simulink model "RobotAndBall"  (R2019b)
settings: Solver=VariableStepAuto  StartTime=0.0  StopTime=30  MaxStep=updateFrequency  RelTol=1e-3
values from neighbouring files (symbols this model uses):
  g = bTraj.GoalOnRight    [Launch_Game_TwoRobots.m]
  pOpponentSidePoint = [2.4;0;0.02]'    [Launch_Game_TwoRobots.m]
  Robot1 = RobotPlayer2(initialQ,TransMat1,DistToTable,'Left')    [Launch_Game_TwoRobots.m]
undefined symbols (not defined in the file or in its folder): Ball, Contact_Forces, currentTime, Environment, Net, Robots, Table, tHit, wayPoints, X, Y, Z
libraries: sm_lib x217, nesl_utility x89, Contact_Forces_Lib x8, robotmaniplib x8, Parts_Lib x6, Multibody_Parts_Lib x2, OpenManipulatorLib x1
(part 3 of 7)

== system RobotAndBall/failTryToPredictTraj ==
  In1 : Inport
  In2 : Inport  Port=2
  Append : MATLAB Function  TreatAsAtomicUnit=on
  Clock : Clock
  MATLAB Function : MATLAB Function  TreatAsAtomicUnit=on
  Subsystem : Subsystem
  Subsystem1 : Subsystem
  Subsystem3 : Subsystem
  Terminator : Terminator
  wires:
  In2/1 -> Append/4(Pnew)
  Append/2(Vout) -> MATLAB Function/2(V), Subsystem3/1(In1)
  MATLAB Function/1(aa) -> Terminator/1
  Clock/1 -> MATLAB Function/4(t)
  Append/3(Nout) -> MATLAB Function/3(N), Subsystem/1(In1)
  Append/1(Pout) -> Subsystem1/1(In1), MATLAB Function/1(P)
  Subsystem3/1(Out1) -> Append/1(V)
  Subsystem/1(Out1) -> Append/5(N)
  Subsystem1/1(Out1) -> Append/3(P)
  In1/1 -> Append/2(Vnew)

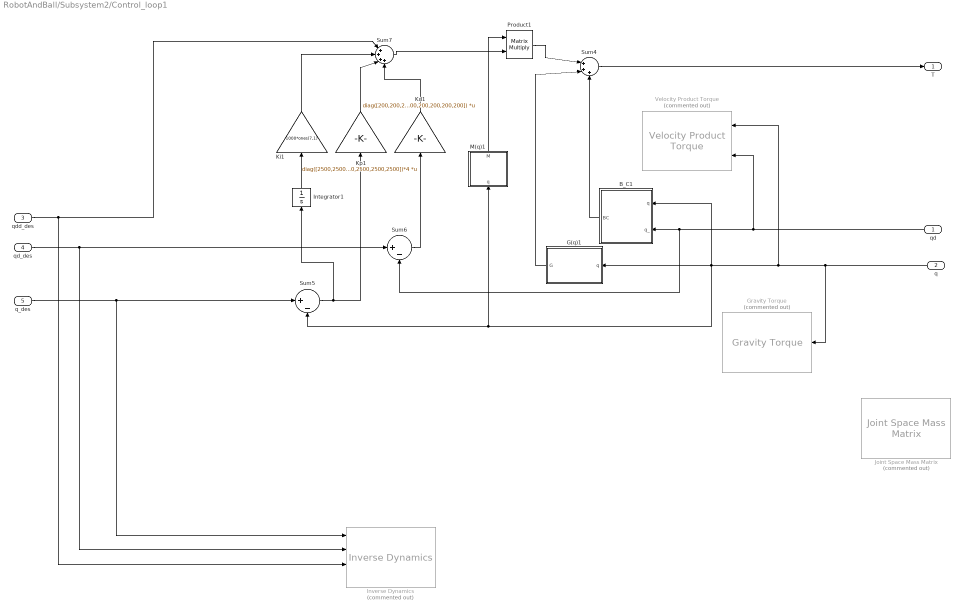
== system RobotAndBall/Subsystem2/Control_loop1 ==
  qd : Inport
  q : Inport  Port=2
  qdd_des : Inport  Port=3
  qd_des : Inport  Port=4
  q_des : Inport  Port=5
  " M(q)1" : MATLAB Function  TreatAsAtomicUnit=on
  B_C1 : MATLAB Function  TreatAsAtomicUnit=on
  G(q)1 : MATLAB Function  TreatAsAtomicUnit=on
  Gravity Torque : robotmaniplib/Gravity Torque  Commented=on  RigidBodyTree=Robot1.RobotModel  SimulateUsing=Code generation
      settings: SourceProductName=Robotics System Toolbox
  Integrator1 : Integrator
  Inverse Dynamics : robotmaniplib/Inverse Dynamics  Commented=on  RigidBodyTree=Robot1.RobotModel  SimulateUsing=Code generation
      settings: SourceProductName=Robotics System Toolbox  SourceProductBaseCode=RO
  Joint Space Mass Matrix : robotmaniplib/Joint Space Mass Matrix  Commented=on  RigidBodyTree=twoJointRigidBodyTree  SimulateUsing=Interpreted execution
      settings: SourceProductName=Robotics System Toolbox
  Kd1 : Gain  Gain=diag([200,200,200,200,200,200,200])  Multiplication=Matrix(K*u) (u vector)
  Ki1 : Gain  Gain=1000*ones(7,1)
  Kp1 : Gain  Gain=diag([2500,2500,2500,2500,2500,2500,2500])*4  Multiplication=Matrix(K*u) (u vector)
  Product1 : Product  Multiplication=Matrix(*)
  Sum4 : Sum  Inputs=|+++
  Sum5 : Sum  Inputs=|+-
  Sum6 : Sum  Inputs=|+-
  Sum7 : Sum  Inputs=|++++
  Velocity Product Torque : robotmaniplib/Velocity Product Torque  Commented=on  RigidBodyTree=Robot1.RobotModel  SimulateUsing=Code generation
      settings: SourceProductName=Robotics System Toolbox  SourceProductBaseCode=RO
  T : Outport
  wires:
  Sum7/1 -> Product1/2
  Kd1/1 -> Sum7/4
  q/1 -> G(q)1/1(q), B_C1/1(q), " M(q)1"/1(q), Sum5/2, Velocity Product Torque/1, Gravity Torque/1
  Sum5/1 -> Kp1/1, Integrator1/1
  Sum6/1 -> Kd1/1
  Ki1/1 -> Sum7/2
  Kp1/1 -> Sum7/3
  " M(q)1"/1(M) -> Product1/1
  Product1/1 -> Sum4/1
  qd_des/1 -> Inverse Dynamics/2, Sum6/1
  Integrator1/1 -> Ki1/1
  qd/1 -> Velocity Product Torque/2, B_C1/2(q_), Sum6/2
  qdd_des/1 -> Inverse Dynamics/3, Sum7/1
  q_des/1 -> Inverse Dynamics/1, Sum5/1
  Sum4/1 -> T/1
  B_C1/1(BC) -> Sum4/3
  G(q)1/1(G) -> Sum4/2

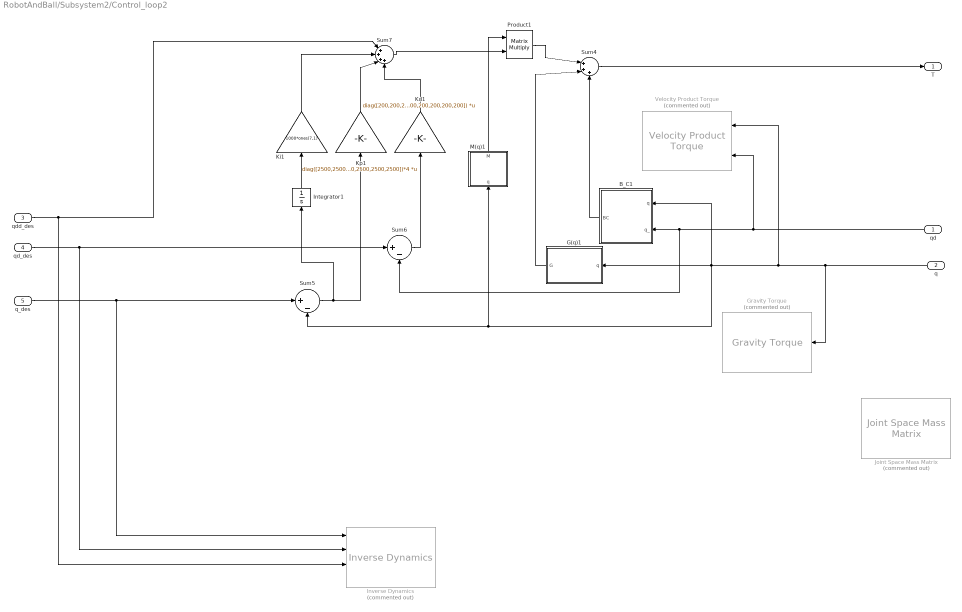
== system RobotAndBall/Subsystem2/Control_loop2 ==
  qd : Inport
  q : Inport  Port=2
  qdd_des : Inport  Port=3
  qd_des : Inport  Port=4
  q_des : Inport  Port=5
  " M(q)1" : MATLAB Function  TreatAsAtomicUnit=on
  B_C1 : MATLAB Function  TreatAsAtomicUnit=on
  G(q)1 : MATLAB Function  TreatAsAtomicUnit=on
  Gravity Torque : robotmaniplib/Gravity Torque  Commented=on  RigidBodyTree=Robot1.RobotModel  SimulateUsing=Code generation
      settings: SourceProductName=Robotics System Toolbox
  Integrator1 : Integrator
  Inverse Dynamics : robotmaniplib/Inverse Dynamics  Commented=on  RigidBodyTree=Robot1.RobotModel  SimulateUsing=Code generation
      settings: SourceProductName=Robotics System Toolbox  SourceProductBaseCode=RO
  Joint Space Mass Matrix : robotmaniplib/Joint Space Mass Matrix  Commented=on  RigidBodyTree=twoJointRigidBodyTree  SimulateUsing=Interpreted execution
      settings: SourceProductName=Robotics System Toolbox
  Kd1 : Gain  Gain=diag([200,200,200,200,200,200,200])  Multiplication=Matrix(K*u) (u vector)
  Ki1 : Gain  Gain=1000*ones(7,1)
  Kp1 : Gain  Gain=diag([2500,2500,2500,2500,2500,2500,2500])*4  Multiplication=Matrix(K*u) (u vector)
  Product1 : Product  Multiplication=Matrix(*)
  Sum4 : Sum  Inputs=|+++
  Sum5 : Sum  Inputs=|+-
  Sum6 : Sum  Inputs=|+-
  Sum7 : Sum  Inputs=|++++
  Velocity Product Torque : robotmaniplib/Velocity Product Torque  Commented=on  RigidBodyTree=Robot1.RobotModel  SimulateUsing=Code generation
      settings: SourceProductName=Robotics System Toolbox  SourceProductBaseCode=RO
  T : Outport
  wires:
  Sum7/1 -> Product1/2
  Kd1/1 -> Sum7/4
  q/1 -> G(q)1/1(q), B_C1/1(q), " M(q)1"/1(q), Sum5/2, Velocity Product Torque/1, Gravity Torque/1
  Sum5/1 -> Kp1/1, Integrator1/1
  Sum6/1 -> Kd1/1
  Ki1/1 -> Sum7/2
  Kp1/1 -> Sum7/3
  " M(q)1"/1(M) -> Product1/1
  Product1/1 -> Sum4/1
  qd_des/1 -> Inverse Dynamics/2, Sum6/1
  Integrator1/1 -> Ki1/1
  qd/1 -> Velocity Product Torque/2, B_C1/2(q_), Sum6/2
  qdd_des/1 -> Inverse Dynamics/3, Sum7/1
  q_des/1 -> Inverse Dynamics/1, Sum5/1
  Sum4/1 -> T/1
  B_C1/1(BC) -> Sum4/3
  G(q)1/1(G) -> Sum4/2

== system RobotAndBall/Subsystem2/Paddle2 ==
  Paddle1 : Parts_Lib/Cylinder  Tag=CustomStyle  Commented=on  cyl_radius=Paddle.Radius  cyl_length=Paddle.thickness  cyl_density=Paddle.density  cyl_color=blue  cyl_opacity=1  cyl_color_custom="[0.7920    0.9900    0.9900]"  mark_radius=[0.75 0.5]  mark_len_factor=1.01  mark_angle=60  mark_color=purple  mark_opacity=1
  Paddle2 : Parts_Lib/Cylinder  Tag=CustomStyle  cyl_radius=Robots.Paddle(1)  cyl_length=Robots.Paddle(2)  cyl_density=Robots.Paddle(3)  cyl_color=blue  cyl_opacity=1  cyl_color_custom="[0.7920    0.9900    0.9900]"  mark_radius=[0.75 0.5]  mark_len_factor=1.01  mark_angle=60  mark_color=purple  mark_opacity=1
      link override Cylinder: Density=cyl_density*0
      link override Vis1: Density=1e-3*0
      link override Vis2: Density=1e-3*0
  Rot1 : sm_lib/Frames and Transforms/Rigid Transform  TranslationMethod=None  TranslationStandardOffset=0  TranslationLengthUnit=m  TranslationStandardAxis=+Z  TranslationCartesianOffset=[0 0 0]  TranslationROffset=0  TranslationROffsetUnits=m  TranslationZOffset=0  TranslationZOffsetUnits=m  TranslationThetaOffset=0  TranslationThetaOffsetUnits=deg  RotationMethod=StandardAxis  RotationAngleUnits=deg  RotationStandardAxis=+Y  RotationAngle=180  RotationArbitraryAxis=[0 0 1]  FollAlignAxisA=+X  BaseAlignAxisA=+Y  FollAlignAxisB=+Y  BaseAlignAxisB=+Z  RotationSequenceAxes=FollowerAxes  RotationSequence=XYX  RotationSequenceAngles=[0 0 0]  RotationSequenceAnglesUnits=deg  RotationMatrix=[1 0 0; 0 1 0; 0 0 1]
      settings: AttributesFormatString=|
      | %<RotationAngle> %<RotationAngleUnits>
      | about %<RotationStandardAxis>
  Rot2 : sm_lib/Frames and Transforms/Rigid Transform  TranslationMethod=None  TranslationStandardOffset=0  TranslationLengthUnit=m  TranslationStandardAxis=+Z  TranslationCartesianOffset=[0 0 0]  TranslationROffset=0  TranslationROffsetUnits=m  TranslationZOffset=0  TranslationZOffsetUnits=m  TranslationThetaOffset=0  TranslationThetaOffsetUnits=deg  RotationMethod=StandardAxis  RotationAngleUnits=deg  RotationStandardAxis=-Y  RotationAngle=90  RotationArbitraryAxis=[0 0 1]  FollAlignAxisA=+X  BaseAlignAxisA=+Y  FollAlignAxisB=+Y  BaseAlignAxisB=+Z  RotationSequenceAxes=FollowerAxes  RotationSequence=XYX  RotationSequenceAngles=[0 0 0]  RotationSequenceAnglesUnits=deg  RotationMatrix=[1 0 0; 0 1 0; 0 0 1]
      settings: AttributesFormatString=|
      | %<RotationAngle> %<RotationAngleUnits>
      | about %<RotationStandardAxis>
  Trans1 : sm_lib/Frames and Transforms/Rigid Transform  TranslationMethod=StandardAxis  TranslationStandardOffset=Robots.Paddle(1)  TranslationLengthUnit=m  TranslationStandardAxis=+Z  TranslationCartesianOffset=[0 0 0]  TranslationROffset=0  TranslationROffsetUnits=m  TranslationZOffset=0  TranslationZOffsetUnits=m  TranslationThetaOffset=0  TranslationThetaOffsetUnits=deg  RotationMethod=None  RotationAngleUnits=deg  RotationStandardAxis=+Z  RotationAngle=0.0  RotationArbitraryAxis=[0 0 1]  FollAlignAxisA=+X  BaseAlignAxisA=+Y  FollAlignAxisB=+Y  BaseAlignAxisB=+Z  RotationSequenceAxes=FollowerAxes  RotationSequence=XYX  RotationSequenceAngles=[0 0 0]  RotationSequenceAnglesUnits=deg  RotationMatrix=[1 0 0; 0 1 0; 0 0 1]
      settings: AttributesFormatString=|
      | %<TranslationStandardOffset> %<TranslationLengthUnit>
      | in %<TranslationStandardAxis>
  B : PMIOPort  Side=Left
  connections:
  Rot1/LConn1 -- B/RConn1
  Trans1/RConn1 -- Rot2/LConn1
  Rot1/RConn1 -- Trans1/LConn1
  Paddle2/LConn1 -- Rot2/RConn1

== system RobotAndBall/Subsystem2/Paddle3 ==
  Paddle1 : Parts_Lib/Cylinder  Tag=CustomStyle  Commented=on  cyl_radius=Paddle.Radius  cyl_length=Paddle.thickness  cyl_density=Paddle.density  cyl_color=blue  cyl_opacity=1  cyl_color_custom="[0.7920    0.9900    0.9900]"  mark_radius=[0.75 0.5]  mark_len_factor=1.01  mark_angle=60  mark_color=purple  mark_opacity=1
  Paddle2 : Parts_Lib/Cylinder  Tag=CustomStyle  cyl_radius=Robots.Paddle(1)  cyl_length=Robots.Paddle(2)  cyl_density=Robots.Paddle(3)  cyl_color=blue  cyl_opacity=1  cyl_color_custom="[0.7920    0.9900    0.9900]"  mark_radius=[0.75 0.5]  mark_len_factor=1.01  mark_angle=60  mark_color=purple  mark_opacity=1
      link override Cylinder: Density=cyl_density*0
      link override Vis1: Density=1e-3*0
      link override Vis2: Density=1e-3*0
  Rot1 : sm_lib/Frames and Transforms/Rigid Transform  TranslationMethod=None  TranslationStandardOffset=0  TranslationLengthUnit=m  TranslationStandardAxis=+Z  TranslationCartesianOffset=[0 0 0]  TranslationROffset=0  TranslationROffsetUnits=m  TranslationZOffset=0  TranslationZOffsetUnits=m  TranslationThetaOffset=0  TranslationThetaOffsetUnits=deg  RotationMethod=StandardAxis  RotationAngleUnits=deg  RotationStandardAxis=+Y  RotationAngle=180  RotationArbitraryAxis=[0 0 1]  FollAlignAxisA=+X  BaseAlignAxisA=+Y  FollAlignAxisB=+Y  BaseAlignAxisB=+Z  RotationSequenceAxes=FollowerAxes  RotationSequence=XYX  RotationSequenceAngles=[0 0 0]  RotationSequenceAnglesUnits=deg  RotationMatrix=[1 0 0; 0 1 0; 0 0 1]
      settings: AttributesFormatString=|
      | %<RotationAngle> %<RotationAngleUnits>
      | about %<RotationStandardAxis>
  Rot2 : sm_lib/Frames and Transforms/Rigid Transform  TranslationMethod=None  TranslationStandardOffset=0  TranslationLengthUnit=m  TranslationStandardAxis=+Z  TranslationCartesianOffset=[0 0 0]  TranslationROffset=0  TranslationROffsetUnits=m  TranslationZOffset=0  TranslationZOffsetUnits=m  TranslationThetaOffset=0  TranslationThetaOffsetUnits=deg  RotationMethod=StandardAxis  RotationAngleUnits=deg  RotationStandardAxis=-Y  RotationAngle=90  RotationArbitraryAxis=[0 0 1]  FollAlignAxisA=+X  BaseAlignAxisA=+Y  FollAlignAxisB=+Y  BaseAlignAxisB=+Z  RotationSequenceAxes=FollowerAxes  RotationSequence=XYX  RotationSequenceAngles=[0 0 0]  RotationSequenceAnglesUnits=deg  RotationMatrix=[1 0 0; 0 1 0; 0 0 1]
      settings: AttributesFormatString=|
      | %<RotationAngle> %<RotationAngleUnits>
      | about %<RotationStandardAxis>
  Trans1 : sm_lib/Frames and Transforms/Rigid Transform  TranslationMethod=StandardAxis  TranslationStandardOffset=Robots.Paddle(1)  TranslationLengthUnit=m  TranslationStandardAxis=+Z  TranslationCartesianOffset=[0 0 0]  TranslationROffset=0  TranslationROffsetUnits=m  TranslationZOffset=0  TranslationZOffsetUnits=m  TranslationThetaOffset=0  TranslationThetaOffsetUnits=deg  RotationMethod=None  RotationAngleUnits=deg  RotationStandardAxis=+Z  RotationAngle=0.0  RotationArbitraryAxis=[0 0 1]  FollAlignAxisA=+X  BaseAlignAxisA=+Y  FollAlignAxisB=+Y  BaseAlignAxisB=+Z  RotationSequenceAxes=FollowerAxes  RotationSequence=XYX  RotationSequenceAngles=[0 0 0]  RotationSequenceAnglesUnits=deg  RotationMatrix=[1 0 0; 0 1 0; 0 0 1]
      settings: AttributesFormatString=|
      | %<TranslationStandardOffset> %<TranslationLengthUnit>
      | in %<TranslationStandardAxis>
  B : PMIOPort  Side=Left
  connections:
  Rot1/LConn1 -- B/RConn1
  Trans1/RConn1 -- Rot2/LConn1
  Rot1/RConn1 -- Trans1/LConn1
  Paddle2/LConn1 -- Rot2/RConn1

== system RobotAndBall/Subsystem2/Paddle4 ==
  Paddle2 : Parts_Lib/Cylinder  Tag=CustomStyle  cyl_radius=Robot1.Paddle(1)  cyl_length=Robot1.Paddle(2)  cyl_density=Robot1.Paddle(3)  cyl_color=red  cyl_opacity=1  cyl_color_custom="[0.7920    0.9900    0.9900]"  mark_radius=[0.75 0.5]  mark_len_factor=1.01  mark_angle=60  mark_color=purple  mark_opacity=1
  Rot1 : sm_lib/Frames and Transforms/Rigid Transform  TranslationMethod=None  TranslationStandardOffset=0  TranslationLengthUnit=m  TranslationStandardAxis=+Z  TranslationCartesianOffset=[0 0 0]  TranslationROffset=0  TranslationROffsetUnits=m  TranslationZOffset=0  TranslationZOffsetUnits=m  TranslationThetaOffset=0  TranslationThetaOffsetUnits=deg  RotationMethod=StandardAxis  RotationAngleUnits=deg  RotationStandardAxis=+Y  RotationAngle=180  RotationArbitraryAxis=[0 0 1]  FollAlignAxisA=+X  BaseAlignAxisA=+Y  FollAlignAxisB=+Y  BaseAlignAxisB=+Z  RotationSequenceAxes=FollowerAxes  RotationSequence=XYX  RotationSequenceAngles=[0 0 0]  RotationSequenceAnglesUnits=deg  RotationMatrix=[1 0 0; 0 1 0; 0 0 1]
      settings: AttributesFormatString=|
      | %<RotationAngle> %<RotationAngleUnits>
      | about %<RotationStandardAxis>
  Rot2 : sm_lib/Frames and Transforms/Rigid Transform  TranslationMethod=None  TranslationStandardOffset=0  TranslationLengthUnit=m  TranslationStandardAxis=+Z  TranslationCartesianOffset=[0 0 0]  TranslationROffset=0  TranslationROffsetUnits=m  TranslationZOffset=0  TranslationZOffsetUnits=m  TranslationThetaOffset=0  TranslationThetaOffsetUnits=deg  RotationMethod=StandardAxis  RotationAngleUnits=deg  RotationStandardAxis=-Y  RotationAngle=90  RotationArbitraryAxis=[0 0 1]  FollAlignAxisA=+X  BaseAlignAxisA=+Y  FollAlignAxisB=+Y  BaseAlignAxisB=+Z  RotationSequenceAxes=FollowerAxes  RotationSequence=XYX  RotationSequenceAngles=[0 0 0]  RotationSequenceAnglesUnits=deg  RotationMatrix=[1 0 0; 0 1 0; 0 0 1]
      settings: AttributesFormatString=|
      | %<RotationAngle> %<RotationAngleUnits>
      | about %<RotationStandardAxis>
  Trans6 : sm_lib/Frames and Transforms/Rigid Transform  TranslationMethod=StandardAxis  TranslationStandardOffset=Robot1.Paddle(1)  TranslationLengthUnit=m  TranslationStandardAxis=+Z  TranslationCartesianOffset=[0 0 0]  TranslationROffset=0  TranslationROffsetUnits=m  TranslationZOffset=0  TranslationZOffsetUnits=m  TranslationThetaOffset=0  TranslationThetaOffsetUnits=deg  RotationMethod=None  RotationAngleUnits=deg  RotationStandardAxis=+Z  RotationAngle=0.0  RotationArbitraryAxis=[0 0 1]  FollAlignAxisA=+X  BaseAlignAxisA=+Y  FollAlignAxisB=+Y  BaseAlignAxisB=+Z  RotationSequenceAxes=FollowerAxes  RotationSequence=XYX  RotationSequenceAngles=[0 0 0]  RotationSequenceAnglesUnits=deg  RotationMatrix=[1 0 0; 0 1 0; 0 0 1]
      settings: AttributesFormatString=|
      | %<TranslationStandardOffset> %<TranslationLengthUnit>
      | in %<TranslationStandardAxis>
  B : PMIOPort  Side=Left
  connections:
  Trans6/RConn1 -- Rot2/LConn1
  Rot1/RConn1 -- Trans6/LConn1
  Paddle2/LConn1 -- Rot2/RConn1
  B/RConn1 -- Rot1/LConn1

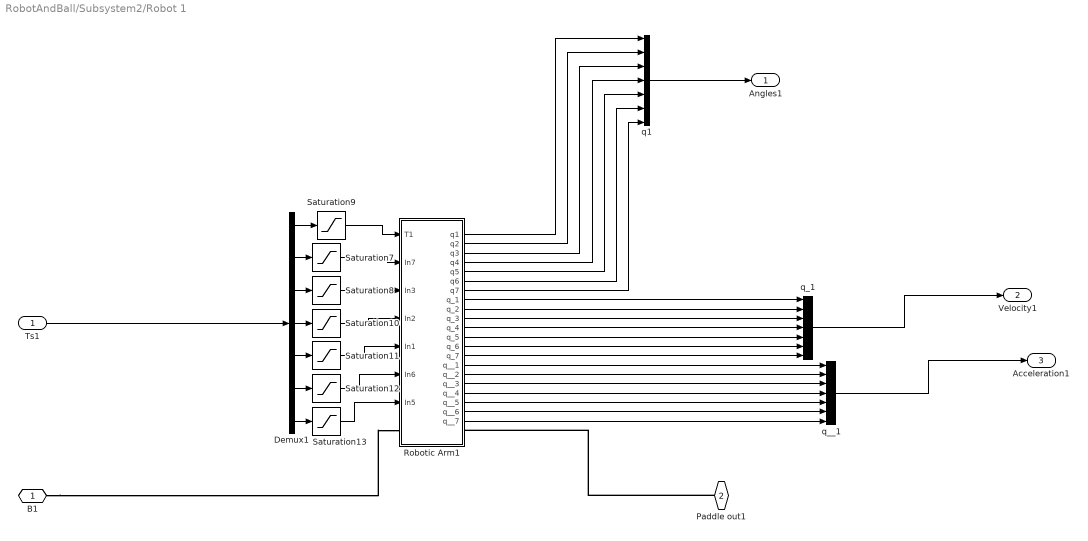
== system RobotAndBall/Subsystem2/Robot 1 ==
  Ts1 : Inport
  Demux1 : Demux  Outputs=7
  Robotic Arm1 : Subsystem
  Saturation10 : Saturate  UpperLimit=110  LowerLimit=-110
  Saturation11 : Saturate  UpperLimit=110  LowerLimit=-110
  Saturation12 : Saturate  UpperLimit=40  LowerLimit=-40
  Saturation13 : Saturate  UpperLimit=40  LowerLimit=-40
  Saturation7 : Saturate  UpperLimit=176  LowerLimit=-176
  Saturation8 : Saturate  UpperLimit=110  LowerLimit=-110
  Saturation9 : Saturate  UpperLimit=176  LowerLimit=-176
  q1 : Mux  Inputs=7
  q_1 : Mux  Inputs=7
  q__1 : Mux  Inputs=7
  B1 : PMIOPort  Side=Left
  Paddle out1 : PMIOPort  Port=2  Side=Right
  Angles1 : Outport
  Velocity1 : Outport  Port=2
  Acceleration1 : Outport  Port=3
  wires:
  q1/1 -> Angles1/1
  q_1/1 -> Velocity1/1
  Robotic Arm1/9(q_2) -> q_1/2
  Saturation13/1 -> Robotic Arm1/7(In5)
  Demux1/2 -> Saturation7/1
  Saturation8/1 -> Robotic Arm1/3(In3)
  Robotic Arm1/6(q6) -> q1/6
  Robotic Arm1/2(q2) -> q1/2
  Demux1/5 -> Saturation11/1
  Saturation7/1 -> Robotic Arm1/2(In7)
  Robotic Arm1/7(q7) -> q1/7
  Robotic Arm1/11(q_4) -> q_1/4
  Demux1/3 -> Saturation8/1
  Demux1/7 -> Saturation13/1
  Demux1/1 -> Saturation9/1
  Robotic Arm1/3(q3) -> q1/3
  Demux1/6 -> Saturation12/1
  Demux1/4 -> Saturation10/1
  Ts1/1 -> Demux1/1
  Saturation11/1 -> Robotic Arm1/5(In1)
  Robotic Arm1/1(q1) -> q1/1
  Robotic Arm1/4(q4) -> q1/4
  Saturation10/1 -> Robotic Arm1/4(In2)
  Robotic Arm1/12(q_5) -> q_1/5
  Robotic Arm1/5(q5) -> q1/5
  Robotic Arm1/8(q_1) -> q_1/1
  Robotic Arm1/13(q_6) -> q_1/6
  Saturation9/1 -> Robotic Arm1/1(T1)
  Robotic Arm1/10(q_3) -> q_1/3
  Robotic Arm1/14(q_7) -> q_1/7
  Saturation12/1 -> Robotic Arm1/6(In6)
  Robotic Arm1/21(q__7) -> q__1/7
  Robotic Arm1/17(q__3) -> q__1/3
  Robotic Arm1/20(q__6) -> q__1/6
  Robotic Arm1/15(q__1) -> q__1/1
  Robotic Arm1/19(q__5) -> q__1/5
  Robotic Arm1/18(q__4) -> q__1/4
  Robotic Arm1/16(q__2) -> q__1/2
  q__1/1 -> Acceleration1/1
  connections:
  B1/RConn1 -- Robotic Arm1/LConn1
  Paddle out1/RConn1 -- Robotic Arm1/RConn1

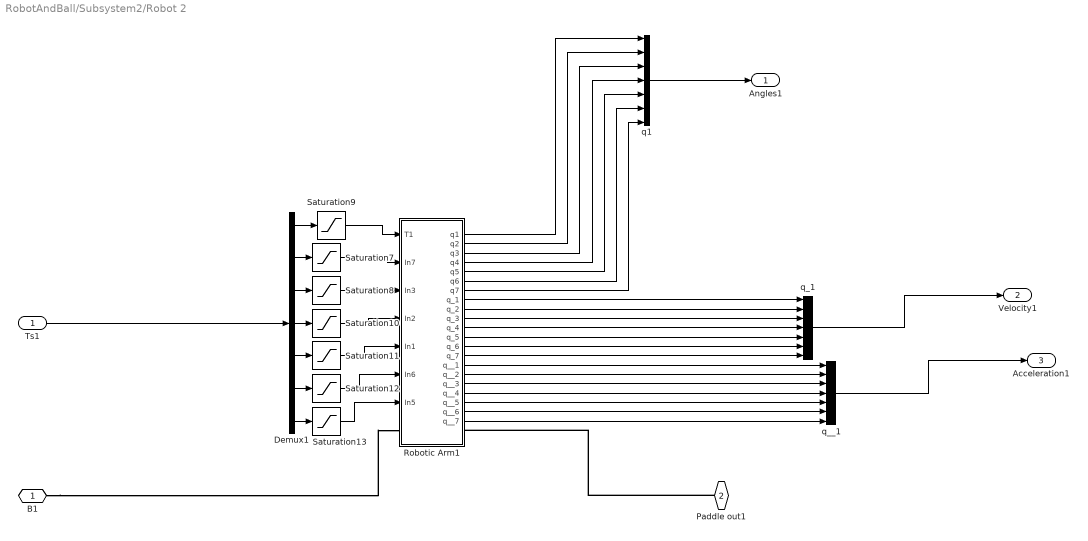
== system RobotAndBall/Subsystem2/Robot 2 ==
  Ts1 : Inport
  Demux1 : Demux  Outputs=7
  Robotic Arm1 : Subsystem
  Saturation10 : Saturate  UpperLimit=110  LowerLimit=-110
  Saturation11 : Saturate  UpperLimit=110  LowerLimit=-110
  Saturation12 : Saturate  UpperLimit=40  LowerLimit=-40
  Saturation13 : Saturate  UpperLimit=40  LowerLimit=-40
  Saturation7 : Saturate  UpperLimit=176  LowerLimit=-176
  Saturation8 : Saturate  UpperLimit=110  LowerLimit=-110
  Saturation9 : Saturate  UpperLimit=176  LowerLimit=-176
  q1 : Mux  Inputs=7
  q_1 : Mux  Inputs=7
  q__1 : Mux  Inputs=7
  B1 : PMIOPort  Side=Left
  Paddle out1 : PMIOPort  Port=2  Side=Right
  Angles1 : Outport
  Velocity1 : Outport  Port=2
  Acceleration1 : Outport  Port=3
  wires:
  q1/1 -> Angles1/1
  q_1/1 -> Velocity1/1
  Robotic Arm1/9(q_2) -> q_1/2
  Saturation13/1 -> Robotic Arm1/7(In5)
  Demux1/2 -> Saturation7/1
  Saturation8/1 -> Robotic Arm1/3(In3)
  Robotic Arm1/6(q6) -> q1/6
  Robotic Arm1/2(q2) -> q1/2
  Demux1/5 -> Saturation11/1
  Saturation7/1 -> Robotic Arm1/2(In7)
  Robotic Arm1/7(q7) -> q1/7
  Robotic Arm1/11(q_4) -> q_1/4
  Demux1/3 -> Saturation8/1
  Demux1/7 -> Saturation13/1
  Demux1/1 -> Saturation9/1
  Robotic Arm1/3(q3) -> q1/3
  Demux1/6 -> Saturation12/1
  Demux1/4 -> Saturation10/1
  Ts1/1 -> Demux1/1
  Saturation11/1 -> Robotic Arm1/5(In1)
  Robotic Arm1/1(q1) -> q1/1
  Robotic Arm1/4(q4) -> q1/4
  Saturation10/1 -> Robotic Arm1/4(In2)
  Robotic Arm1/12(q_5) -> q_1/5
  Robotic Arm1/5(q5) -> q1/5
  Robotic Arm1/8(q_1) -> q_1/1
  Robotic Arm1/13(q_6) -> q_1/6
  Saturation9/1 -> Robotic Arm1/1(T1)
  Robotic Arm1/10(q_3) -> q_1/3
  Robotic Arm1/14(q_7) -> q_1/7
  Saturation12/1 -> Robotic Arm1/6(In6)
  Robotic Arm1/21(q__7) -> q__1/7
  Robotic Arm1/17(q__3) -> q__1/3
  Robotic Arm1/20(q__6) -> q__1/6
  Robotic Arm1/15(q__1) -> q__1/1
  Robotic Arm1/19(q__5) -> q__1/5
  Robotic Arm1/18(q__4) -> q__1/4
  Robotic Arm1/16(q__2) -> q__1/2
  q__1/1 -> Acceleration1/1
  connections:
  B1/RConn1 -- Robotic Arm1/LConn1
  Paddle out1/RConn1 -- Robotic Arm1/RConn1

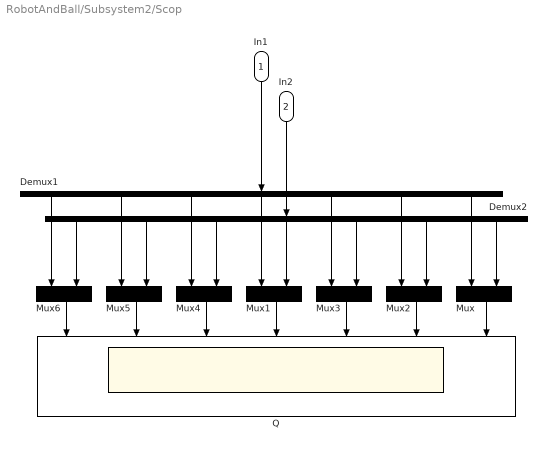
== system RobotAndBall/Subsystem2/Scop ==
  In1 : Inport
  In2 : Inport  Port=2
  Demux1 : Demux  Outputs=7
  Demux2 : Demux  Outputs=7
  Mux{,1..6} (7 alike) : Mux  Inputs=2
  Q : Scope  NumInputPorts=7
  wires:
  In2/1 -> Demux2/1
  Mux/1 -> Q/7
  Mux2/1 -> Q/6
  Mux3/1 -> Q/5
  Mux1/1 -> Q/4
  Mux4/1 -> Q/3
  Mux5/1 -> Q/2
  Mux6/1 -> Q/1
  Demux2/7 -> Mux/2
  Demux2/1 -> Mux6/2
  Demux2/6 -> Mux2/2
  Demux2/5 -> Mux3/2
  Demux2/4 -> Mux1/2
  Demux2/3 -> Mux4/2
  Demux2/2 -> Mux5/2
  Demux1/7 -> Mux/1
  Demux1/6 -> Mux2/1
  Demux1/5 -> Mux3/1
  Demux1/4 -> Mux1/1
  Demux1/3 -> Mux4/1
  Demux1/2 -> Mux5/1
  Demux1/1 -> Mux6/1
  In1/1 -> Demux1/1

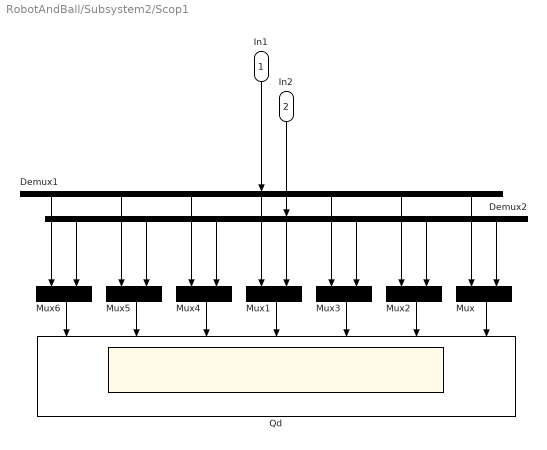
== system RobotAndBall/Subsystem2/Scop1 ==
  In1 : Inport
  In2 : Inport  Port=2
  Demux1 : Demux  Outputs=7
  Demux2 : Demux  Outputs=7
  Mux{,1..6} (7 alike) : Mux  Inputs=2
  Qd : Scope  NumInputPorts=7
  wires:
  In1/1 -> Demux1/1
  Demux1/1 -> Mux6/1
  Demux1/2 -> Mux5/1
  Demux1/3 -> Mux4/1
  Demux1/4 -> Mux1/1
  Demux1/5 -> Mux3/1
  Demux1/6 -> Mux2/1
  Demux1/7 -> Mux/1
  Demux2/2 -> Mux5/2
  Demux2/3 -> Mux4/2
  Demux2/4 -> Mux1/2
  Demux2/5 -> Mux3/2
  Demux2/6 -> Mux2/2
  Demux2/1 -> Mux6/2
  Demux2/7 -> Mux/2
  Mux6/1 -> Qd/1
  Mux5/1 -> Qd/2
  Mux4/1 -> Qd/3
  Mux1/1 -> Qd/4
  Mux3/1 -> Qd/5
  Mux2/1 -> Qd/6
  Mux/1 -> Qd/7
  In2/1 -> Demux2/1

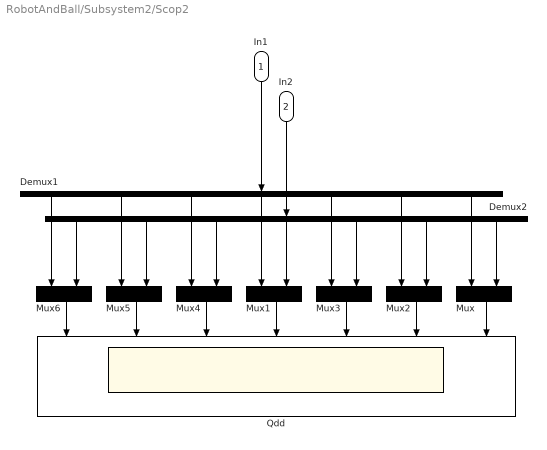
== system RobotAndBall/Subsystem2/Scop2 ==
  In1 : Inport
  In2 : Inport  Port=2
  Demux1 : Demux  Outputs=7
  Demux2 : Demux  Outputs=7
  Mux{,1..6} (7 alike) : Mux  Inputs=2
  Qdd : Scope  NumInputPorts=7
  wires:
  In2/1 -> Demux2/1
  Mux/1 -> Qdd/7
  Mux2/1 -> Qdd/6
  Mux3/1 -> Qdd/5
  Mux1/1 -> Qdd/4
  Mux4/1 -> Qdd/3
  Mux5/1 -> Qdd/2
  Mux6/1 -> Qdd/1
  Demux2/7 -> Mux/2
  Demux2/1 -> Mux6/2
  Demux2/6 -> Mux2/2
  Demux2/5 -> Mux3/2
  Demux2/4 -> Mux1/2
  Demux2/3 -> Mux4/2
  Demux2/2 -> Mux5/2
  Demux1/7 -> Mux/1
  Demux1/6 -> Mux2/1
  Demux1/5 -> Mux3/1
  Demux1/4 -> Mux1/1
  Demux1/3 -> Mux4/1
  Demux1/2 -> Mux5/1
  Demux1/1 -> Mux6/1
  In1/1 -> Demux1/1

== system RobotAndBall/Subsystem2/Scop3 ==
  In1 : Inport
  In2 : Inport  Port=2
  Demux1 : Demux  Outputs=7
  Demux2 : Demux  Outputs=7
  Mux{,1..6} (7 alike) : Mux  Inputs=2
  Q : Scope  NumInputPorts=7
  wires:
  In2/1 -> Demux2/1
  Mux/1 -> Q/7
  Mux2/1 -> Q/6
  Mux3/1 -> Q/5
  Mux1/1 -> Q/4
  Mux4/1 -> Q/3
  Mux5/1 -> Q/2
  Mux6/1 -> Q/1
  Demux2/7 -> Mux/2
  Demux2/1 -> Mux6/2
  Demux2/6 -> Mux2/2
  Demux2/5 -> Mux3/2
  Demux2/4 -> Mux1/2
  Demux2/3 -> Mux4/2
  Demux2/2 -> Mux5/2
  Demux1/7 -> Mux/1
  Demux1/6 -> Mux2/1
  Demux1/5 -> Mux3/1
  Demux1/4 -> Mux1/1
  Demux1/3 -> Mux4/1
  Demux1/2 -> Mux5/1
  Demux1/1 -> Mux6/1
  In1/1 -> Demux1/1

== system RobotAndBall/Subsystem2/Scop4 ==
  In1 : Inport
  In2 : Inport  Port=2
  Demux1 : Demux  Outputs=7
  Demux2 : Demux  Outputs=7
  Mux{,1..6} (7 alike) : Mux  Inputs=2
  Qd : Scope  NumInputPorts=7
  wires:
  In1/1 -> Demux1/1
  Demux1/1 -> Mux6/1
  Demux1/2 -> Mux5/1
  Demux1/3 -> Mux4/1
  Demux1/4 -> Mux1/1
  Demux1/5 -> Mux3/1
  Demux1/6 -> Mux2/1
  Demux1/7 -> Mux/1
  Demux2/2 -> Mux5/2
  Demux2/3 -> Mux4/2
  Demux2/4 -> Mux1/2
  Demux2/5 -> Mux3/2
  Demux2/6 -> Mux2/2
  Demux2/1 -> Mux6/2
  Demux2/7 -> Mux/2
  Mux6/1 -> Qd/1
  Mux5/1 -> Qd/2
  Mux4/1 -> Qd/3
  Mux1/1 -> Qd/4
  Mux3/1 -> Qd/5
  Mux2/1 -> Qd/6
  Mux/1 -> Qd/7
  In2/1 -> Demux2/1

== system RobotAndBall/Subsystem2/Scop5 ==
  In1 : Inport
  In2 : Inport  Port=2
  Demux1 : Demux  Outputs=7
  Demux2 : Demux  Outputs=7
  Mux{,1..6} (7 alike) : Mux  Inputs=2
  Qdd : Scope  NumInputPorts=7
  wires:
  In2/1 -> Demux2/1
  Mux/1 -> Qdd/7
  Mux2/1 -> Qdd/6
  Mux3/1 -> Qdd/5
  Mux1/1 -> Qdd/4
  Mux4/1 -> Qdd/3
  Mux5/1 -> Qdd/2
  Mux6/1 -> Qdd/1
  Demux2/7 -> Mux/2
  Demux2/1 -> Mux6/2
  Demux2/6 -> Mux2/2
  Demux2/5 -> Mux3/2
  Demux2/4 -> Mux1/2
  Demux2/3 -> Mux4/2
  Demux2/2 -> Mux5/2
  Demux1/7 -> Mux/1
  Demux1/6 -> Mux2/1
  Demux1/5 -> Mux3/1
  Demux1/4 -> Mux1/1
  Demux1/3 -> Mux4/1
  Demux1/2 -> Mux5/1
  Demux1/1 -> Mux6/1
  In1/1 -> Demux1/1

== system RobotAndBall/Subsystem2/Subsystem1 ==
  Table : sm_lib/Body Elements/Brick Solid  GraphicAmbientColor=[0.15 0.15 0.15 1.0]  BasedOnType=Density  BrickDimensions=[Table.Dimensions(1) Table.Dimensions(2) Table.Dimensions(3)]  BrickDimensionUnits=m  CenterOfMass=[0 0 0]  CenterOfMassUnits=m  GraphicDiffuseColor=[0.0 0.4 0.4]  Density=Table.Dimensions(4)  DensityUnits=kg/(m^3)  DoExposeReferenceFrame=on  GraphicEmissiveColor=[0.0 0.0 0.0 1.0]  ExportEntireGeometry=off  SerializedFrames=<Frames/>  MarkerShape=Sphere  MarkerSize=10  GraphicType=FromGeometry  InertiaType=CalculateFromGeometry  Mass=1  MassUnits=kg  MomentsOfInertia=[1 1 1]  MomentsOfInertiaUnits=kg*m^2  GraphicOpacity=1.0  ProductsOfInertia=[0 0 0]  ProductsOfInertiaUnits=kg*m^2  GraphicShininess=75  GraphicSpecularColor=[0.5 0.5 0.5 1.0]  GraphicVisPropType=SimpleVisualProperties
  Trans Table 3 : sm_lib/Frames and Transforms/Rigid Transform  TranslationMethod=StandardAxis  TranslationStandardOffset=0*(Table.Height)-Table.Dimensions(3)/2  TranslationLengthUnit=m  TranslationStandardAxis=+Z  TranslationCartesianOffset=[0 0 0]  TranslationROffset=0  TranslationROffsetUnits=m  TranslationZOffset=0  TranslationZOffsetUnits=m  TranslationThetaOffset=0  TranslationThetaOffsetUnits=deg  RotationMethod=None  RotationAngleUnits=deg  RotationStandardAxis=+Z  RotationAngle=0.0  RotationArbitraryAxis=[0 0 1]  FollAlignAxisA=+X  BaseAlignAxisA=+Y  FollAlignAxisB=+Y  BaseAlignAxisB=+Z  RotationSequenceAxes=FollowerAxes  RotationSequence=XYX  RotationSequenceAngles=[0 0 0]  RotationSequenceAnglesUnits=deg  RotationMatrix=[1 0 0; 0 1 0; 0 0 1]
      settings: AttributesFormatString=|
      | %<TranslationStandardOffset> %<TranslationLengthUnit>
      | in %<TranslationStandardAxis>
  In : PMIOPort  Side=Left
  Bottom : PMIOPort  Port=2  Side=Right
  Center_Table : PMIOPort  Port=3  Side=Right
  connections:
  Center_Table/RConn1 -- Trans Table 3/RConn1 -- Table/RConn1
  Bottom/RConn1 -- In/RConn1 -- Trans Table 3/LConn1

== system RobotAndBall/Subsystem2/Third_deg_traj ==
  Clock : Clock
  Constant : Constant  Value=Robot1.qHit
  MATLAB Function3 : MATLAB Function  TreatAsAtomicUnit=on
  Tf : Constant  Value=[1,1,1,1,1,1,1]*tHit
  Ti : Constant  Value=ones(7,1)*0.07
  qi : Constant  Value=Robot1.initialQ  OutDataTypeStr=double
  q__ : Outport
  q_ : Outport  Port=2
  q : Outport  Port=3
  wires:
  Ti/1 -> MATLAB Function3/2(Ti)
  Tf/1 -> MATLAB Function3/3(Tf)
  Constant/1 -> MATLAB Function3/5(qf)
  MATLAB Function3/3(q) -> q/1
  Clock/1 -> MATLAB Function3/1(t)
  qi/1 -> MATLAB Function3/4(qi)
  MATLAB Function3/1(q__) -> q__/1
  MATLAB Function3/2(q_) -> q_/1

== system RobotAndBall/Subsystem2/Waypoint Visuals ==
  Trajectory Spline : sm_lib/Curves and Surfaces/Spline  GraphicAmbientColor=[0.15 0.15 0.15 1.0]  GraphicDiffuseColor=splineColor  DataPoints=splinePoints  DataPointsUnits=m  GraphicEmissiveColor=[0.0 0.0 0.0 1.0]  EndConditionType=Natural  MarkerShape=Sphere  MarkerSize=10  GraphicType=FromGeometry  GraphicOpacity=1.0  GraphicShininess=75  GraphicSpecularColor=[0.5 0.5 0.5 1.0]  GraphicVisPropType=SimpleVisualProperties
      settings: SourceProductName=Simscape Multibody
  W : PMIOPort  Side=Left
  connections:
  Trajectory Spline/LConn1 -- W/RConn1
  ?
  ?
  ?
  ?

== system RobotAndBall/failTryToPredictTraj/Subsystem ==
  In1 : Inport
  Clock : Clock
  Constant : Constant  Value=0
  Delay1 : Delay
  Switch : Switch  Threshold=0.001
  Out1 : Outport
  wires:
  Delay1/1 -> Switch/3
  Clock/1 -> Switch/2
  Constant/1 -> Switch/1
  In1/1 -> Delay1/1
  Switch/1 -> Out1/1

== system RobotAndBall/failTryToPredictTraj/Subsystem1 ==
  In1 : Inport
  Clock1 : Clock
  Constant1 : Constant  Value=zeros(1000,3)
  Delay : Delay
  Switch1 : Switch  Threshold=0.001
  Out1 : Outport
  wires:
  Switch1/1 -> Out1/1
  Delay/1 -> Switch1/3
  Constant1/1 -> Switch1/1
  Clock1/1 -> Switch1/2
  In1/1 -> Delay/1

== system RobotAndBall/failTryToPredictTraj/Subsystem3 ==
  In1 : Inport
  Clock1 : Clock
  Constant1 : Constant  Value=zeros(1000,3)
  Delay : Delay
  Switch1 : Switch  Threshold=0.001
  Out1 : Outport
  wires:
  Switch1/1 -> Out1/1
  Delay/1 -> Switch1/3
  Constant1/1 -> Switch1/1
  Clock1/1 -> Switch1/2
  In1/1 -> Delay/1
